simulink model "bola_saltitonaP12"  (R2015a)
settings: Solver=ode3  StartTime=0.0  StopTime=20  FixedStep=1e-4  RelTol=1e-3
libraries: simulink x1
settings Model: Creator=ModSim  LastModifiedBy=Alunos
settings DataIOCC: InspectSignalLogs=on
settings DebuggingCC: MaxConsecutiveZCsMsg=none

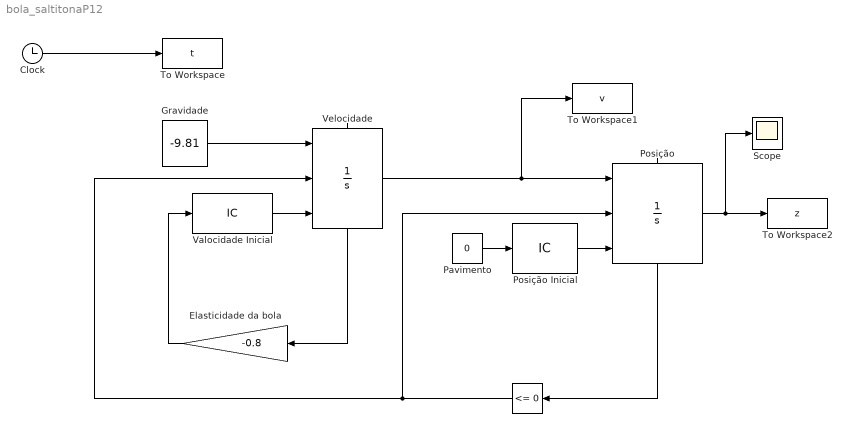
== system bola_saltitonaP12 ==
  " " : simulink/Logic and Bit Operations/Compare To Zero  relop=<=  OutDataTypeStr=boolean
  " Posição" : Integrator  ExternalReset=rising  InitialConditionSource=external  LimitOutput=on  LowerSaturationLimit=0  ShowStatePort=on
  Clock : Clock
  Elasticidade da bola : Gain  Gain=-0.8
  Gravidade : Constant  Value=-9.81
  Pavimento : Constant  Value=0
  Posição Inicial : InitialCondition  Value=10
  Scope : Scope
  To Workspace : ToWorkspace  VariableName=t  SampleTime=-1
  To Workspace1 : ToWorkspace  VariableName=v  SampleTime=-1
  To Workspace2 : ToWorkspace  VariableName=z  SampleTime=-1
  Valocidade Inicial : InitialCondition  Value=15
  Velocidade : Integrator  ExternalReset=rising  InitialConditionSource=external  ShowStatePort=on
  wires:
  Valocidade Inicial/1 -> Velocidade/3
  Velocidade/State -> Elasticidade da bola/1
  " "/1 -> Velocidade/2, " Posição"/2
  Clock/1 -> To Workspace/1
  Posição Inicial/1 -> " Posição"/3
  Pavimento/1 -> Posição Inicial/1
  Elasticidade da bola/1 -> Valocidade Inicial/1
  " Posição"/1 -> To Workspace2/1, Scope/1
  Velocidade/1 -> " Posição"/1, To Workspace1/1
  Gravidade/1 -> Velocidade/1
  " Posição"/State -> " "/1
